simulink model "Simulator"  (R2023b)
settings: Solver=ode5  StartTime=0.0  StopTime=time.value/15/24  FixedStep=clock.sampleTime.value  RelTol=1e-11  AbsTol=1e-12
undefined symbols (not defined in the file or in its folder): aging_clock, attitude, bias_clock, bias_gyro, chi2inv, clock, drift_clock, Environment, IMU, IMU_filter, Propagation, R_sensor2body, starTracker, vb, vm, x0, xb, xm
libraries: matrix_library x11, sensors_subsystems x4, nav_lib x3, aerolibutil x2, dyn_lib x1, simulink x1
settings Model: DataDictionary=SimulationDict.sldd  EnableAccessToBaseWorkspace=off  SimulationMode=accelerator  Creator=brent  LastModifiedBy=brent
settings SolverCC: MinimalZcImpactIntegration=on
settings DebuggingCC: ReadBeforeWriteMsg=DisableAll  WriteAfterWriteMsg=DisableAll  WriteAfterReadMsg=DisableAll  MultiTaskDSMMsg=none
settings ModelReferenceCC: UpdateModelReferenceTargets=IfOutOfDate
settings SFSimCC: SFSimEcho=off
settings RTWCC: BuildConfiguration=Faster Runs

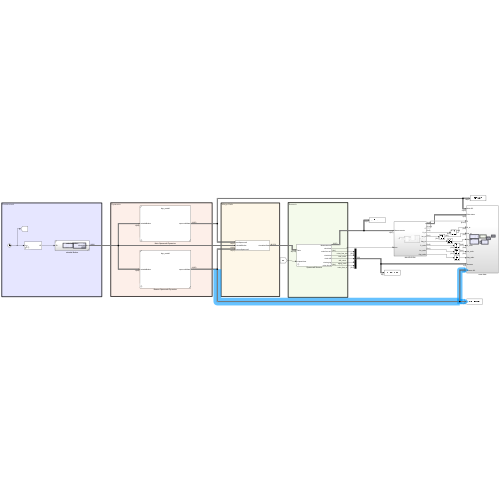
[thumbnail: Simulink's stored preview of the top-level diagram]
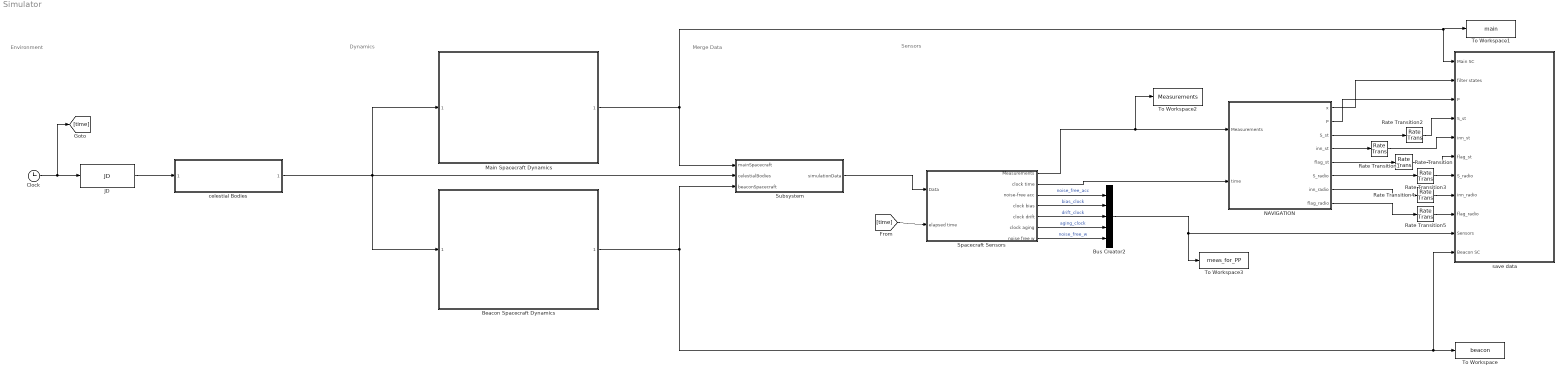
== system Simulator ==
  note: Sensors
  note: Merge Data
  note: Dynamics
  note: Environment
  Beacon Spacecraft Dynamics : Subsystem  ReferencedSubsystem=dyn_model  Environment=Environment  Spacecraft=BeaconSpacecraft  sc_type="\"beacon\""
  Bus Creator2 : BusCreator  Inputs=5
  Clock : Clock
  JD : dyn_lib/JD  year=Environment.Date.year  month=Environment.Date.month  day=Environment.Date.day  hour=Environment.Date.hour  min=Environment.Date.min  sec=Environment.Date.sec
      settings: SourceProductName=Dynamics library
  Main Spacecraft Dynamics : Subsystem  ReferencedSubsystem=dyn_model  Environment=Environment  Spacecraft=MainSpacecraft  sc_type="\"main\""
  NAVIGATION : Subsystem
  Rate Transition{,1..5} (6 alike) : RateTransition  OutPortSampleTime=1/Propagation.lf.value
  Spacecraft Sensors : Subsystem
      mask DialogControl DescGroupVar Prompt: Main spacecraft sensors
  Subsystem : Subsystem
  To Workspace : ToWorkspace  VariableName=beacon  SaveFormat=Timeseries  SampleTime=-1
  To Workspace1 : ToWorkspace  VariableName=main  SaveFormat=Timeseries  SampleTime=-1
  To Workspace2 : ToWorkspace  VariableName=Measurements  SaveFormat=Timeseries  SampleTime=-1
  To Workspace3 : ToWorkspace  VariableName=meas_for_PP  SaveFormat=Timeseries  SampleTime=-1
  celestial Bodies : Subsystem  ReferencedSubsystem=celestialBodies
      settings: PermitHierarchicalResolution=None
  save data : Subsystem
  wires:
  JD/1 -> celestial Bodies/1
  Clock/1 -> [time], JD/1
  celestial Bodies/1 -> Main Spacecraft Dynamics/1, Subsystem/2(celestialBodies), Beacon Spacecraft Dynamics/1
  Subsystem/1(simulationData) -> Spacecraft Sensors/1(Data)
  [time] -> Spacecraft Sensors/2(elapsed time)
  NAVIGATION/1(x) -> save data/2(filter states)
  Spacecraft Sensors/2(clock time) -> NAVIGATION/2(time)
  Spacecraft Sensors/1(Measurements) -> To Workspace2/1, NAVIGATION/1(Measurements)
  Main Spacecraft Dynamics/1 -> Subsystem/1(mainSpacecraft), save data/1(Main SC), To Workspace1/1
  Beacon Spacecraft Dynamics/1 -> To Workspace/1, save data/11(Beacon SC), Subsystem/3(beaconSpacecraft)
  Spacecraft Sensors/4(clock bias) -> Bus Creator2/2  "bias_clock"
  Spacecraft Sensors/5(clock drift) -> Bus Creator2/3  "drift_clock"
  Spacecraft Sensors/3(noise-free acc) -> Bus Creator2/1  "noise_free_acc"
  Spacecraft Sensors/6(clock aging) -> Bus Creator2/4  "aging_clock"
  Spacecraft Sensors/7(noise free w) -> Bus Creator2/5  "noise_free_w"
  Bus Creator2/1 -> To Workspace3/1, save data/10(Sensors)
  NAVIGATION/2(P) -> save data/3(P)
  NAVIGATION/3(S_st) -> Rate Transition2/1
  NAVIGATION/4(inn_st) -> Rate Transition1/1
  NAVIGATION/5(flag_st) -> Rate Transition/1
  Rate Transition/1 -> save data/6(flag_st)
  Rate Transition1/1 -> save data/5(inn_st)
  Rate Transition2/1 -> save data/4(S_st)
  NAVIGATION/6(S_radio) -> Rate Transition3/1
  NAVIGATION/7(inn_radio) -> Rate Transition4/1
  NAVIGATION/8(flag_radio) -> Rate Transition5/1
  Rate Transition3/1 -> save data/7(S_radio)
  Rate Transition4/1 -> save data/8(inn_radio)
  Rate Transition5/1 -> save data/9(flag_radio)

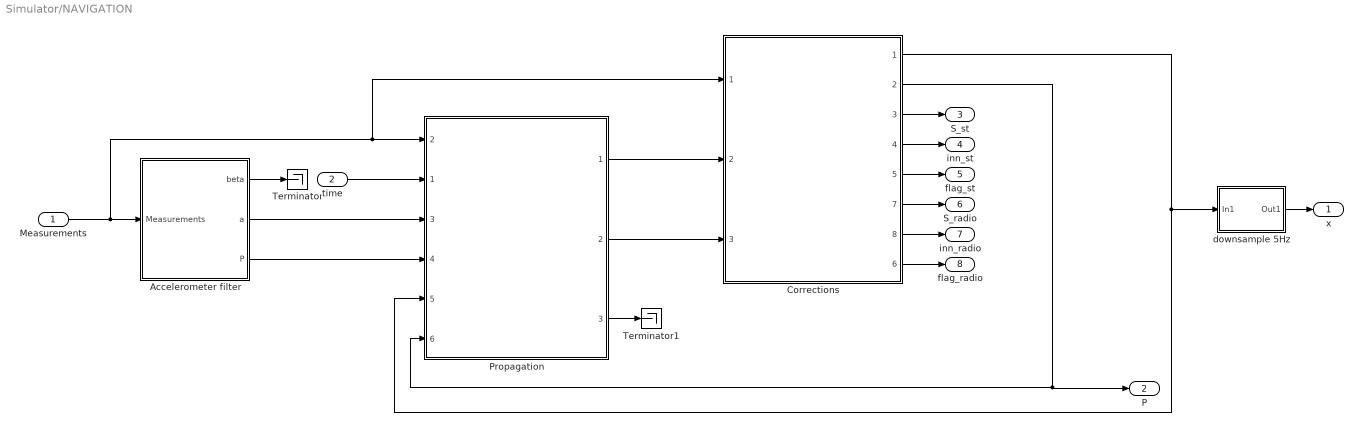
== system Simulator/NAVIGATION ==
  Measurements : Inport
  time : Inport  Port=2
  Accelerometer filter : Subsystem
  Corrections : Subsystem  SystemSampleTime=1/Propagation.lf.value  ReferencedSubsystem=Corrections
      settings: PortSchema="{\"entries\":[{\"content\":{\"sides\":[{\"content\":{\"connectorIds\":[\"In1\",\"In2\",\"In3\"]},\"type\":\"ConnectorPlacement.EquallySpacedRectSide\",\"uuid\":\"4a0e20b6-6862-4fa1-a2e9-6e1d8bf74bd7\"},{\"content\":{\"connectorIds\":[\"Out1\",\"Out2\",\"Out3\",\"Out4\",\"Out5\",\"Out7\",\"Out8\",\"Out6\"],\"side\":\"RIGHT\"},\"type\":\"ConnectorPlacement.EquallySpacedRectSide\",\"uuid\":\"f2385953-66e1-45ae-9533-3c9604da3d88\"},{\"content\":{\"side\":\"TOP\"},\"type\":\"ConnectorPlacement.EquallySpacedRectSide\",\"uuid\":\"afdba90b-0ddf-41f8-b327-cae45893fc5e\"}]},\"type\":\"ConnectorPlacement.EquallySpacedConnector\",\"uuid\":\"034f2023-7f19-4627-93e0-5347c716ea57\"}],\"packageUris\":[\"http://schema.mathworks.com/mf0/Connector/R2020b\"],\"version\":\"1.0\"}"
  Propagation : Subsystem  ReferencedSubsystem=propagation
      settings: PortSchema="{\"entries\":[{\"content\":{\"sides\":[{\"content\":{\"connectorIds\":[\"In2\",\"In1\",\"In3\",\"In4\",\"In5\",\"In6\"]},\"type\":\"ConnectorPlacement.EquallySpacedRectSide\",\"uuid\":\"bbcb9a4b-74e9-4951-92cf-711ba847ce16\"},{\"content\":{\"connectorIds\":[\"Out1\",\"Out2\",\"Out3\"],\"side\":\"RIGHT\"},\"type\":\"ConnectorPlacement.EquallySpacedRectSide\",\"uuid\":\"3c0c2903-3498-4d45-863b-5de13beed929\"},{\"content\":{\"side\":\"TOP\"},\"type\":\"ConnectorPlacement.EquallySpacedRectSide\",\"uuid\":\"36c2c2d5-e434-425c-9c60-e059bfa56cb3\"}]},\"type\":\"ConnectorPlacement.EquallySpacedConnector\",\"uuid\":\"92b99c71-176e-44fa-97a0-fffc1d5455e4\"}],\"packageUris\":[\"http://schema.mathworks.com/mf0/Connector/R2020b\"],\"version\":\"1.0\"}"
  Terminator : Terminator
  Terminator1 : Terminator
  downsample 5Hz : Subsystem  TreatAsAtomicUnit=on  SystemSampleTime=1/Propagation.lf.value
  x : Outport
  P : Outport  Port=2
  S_st : Outport  Port=3
  inn_st : Outport  Port=4
  flag_st : Outport  Port=5
  S_radio : Outport  Port=6
  inn_radio : Outport  Port=7
  flag_radio : Outport  Port=8
  wires:
  time/1 -> Propagation/1
  Propagation/1 -> Corrections/2
  Propagation/2 -> Corrections/3
  Corrections/2 -> P/1, Propagation/6
  Measurements/1 -> Accelerometer filter/1(Measurements), Corrections/1, Propagation/2
  Corrections/1 -> downsample 5Hz/1(In1), Propagation/5
  Propagation/3 -> Terminator1/1
  downsample 5Hz/1(Out1) -> x/1
  Accelerometer filter/1(beta) -> Terminator/1
  Accelerometer filter/2(a) -> Propagation/3
  Accelerometer filter/3(P) -> Propagation/4
  Corrections/3 -> S_st/1
  Corrections/5 -> flag_st/1
  Corrections/4 -> inn_st/1
  Corrections/7 -> S_radio/1
  Corrections/8 -> inn_radio/1
  Corrections/6 -> flag_radio/1

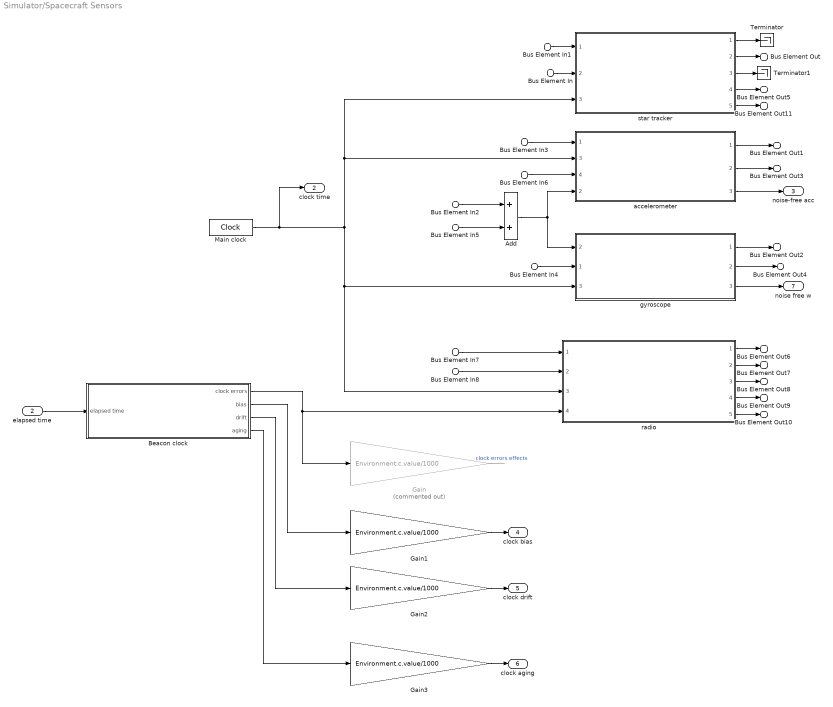
== system Simulator/Spacecraft Sensors ==
  Bus Element In1 : Inport  PortName=Data  Element=celestialBodies
  Bus Element In8 : Inport  PortName=Data  Element=beaconSpacecraft.x
  Bus Element In : Inport  PortName=Data  Element=mainSpacecraft
  Bus Element In7 : Inport  PortName=Data  Element=mainSpacecraft.x
  Bus Element In3 : Inport  PortName=Data  Element=mainSpacecraft.w
  Bus Element In4 : Inport  PortName=Data  Element=mainSpacecraft.w
  Bus Element In6 : Inport  PortName=Data  Element=mainSpacecraft.q
  Bus Element In2 : Inport  PortName=Data  Element=mainSpacecraft.a.srp
  Bus Element In5 : Inport  PortName=Data  Element=mainSpacecraft.a.thrust
  elapsed time : Inport  Port=2
  " Beacon clock" : Subsystem  TreatAsAtomicUnit=on  SystemSampleTime=clock.sampleTime.value
  Add : Sum
  Gain : Gain  Commented=on  Gain=Environment.c.value/1000
  Gain1 : Gain  Gain=Environment.c.value/1000
  Gain2 : Gain  Gain=Environment.c.value/1000
  Gain3 : Gain  Gain=Environment.c.value/1000
  Main clock : DigitalClock  SampleTime=clock.sampleTime.value
  Terminator : Terminator
  Terminator1 : Terminator
  accelerometer : Subsystem  TreatAsAtomicUnit=on  SystemSampleTime=IMU.accelerometer.sampleTime.value  ReferencedSubsystem=accelerometer
      settings: PortSchema="{\"entries\":[{\"content\":{\"sides\":[{\"content\":{\"connectorIds\":[\"In1\",\"In3\",\"In4\",\"In2\"]},\"type\":\"ConnectorPlacement.EquallySpacedRectSide\",\"uuid\":\"f690aca1-0f02-47fc-8596-4493e25f285c\"},{\"content\":{\"connectorIds\":[\"Out1\",\"Out2\",\"Out3\"],\"side\":\"RIGHT\"},\"type\":\"ConnectorPlacement.EquallySpacedRectSide\",\"uuid\":\"ecd25334-8389-4aa4-af3e-65bbeaac2b4b\"},{\"content\":{\"side\":\"TOP\"},\"type\":\"ConnectorPlacement.EquallySpacedRectSide\",\"uuid\":\"886a7907-fe4b-4c0c-bdd8-227e17cf6450\"}]},\"type\":\"ConnectorPlacement.EquallySpacedConnector\",\"uuid\":\"5845c284-1d3d-44f6-9189-c640147e7586\"}],\"packageUris\":[\"http://schema.mathworks.com/mf0/Connector/R2020b\"],\"version\":\"1.0\"}"
  gyroscope : Subsystem  TreatAsAtomicUnit=on  SystemSampleTime=IMU.gyroscope.sampleTime.value  ReferencedSubsystem=gyroscope
      settings: PortSchema="{\"entries\":[{\"content\":{\"sides\":[{\"content\":{\"connectorIds\":[\"In2\",\"In1\",\"In3\"]},\"type\":\"ConnectorPlacement.EquallySpacedRectSide\",\"uuid\":\"a73d9eac-a576-4678-b54d-8c746de67cbf\"},{\"content\":{\"connectorIds\":[\"Out1\",\"Out2\",\"Out3\"],\"side\":\"RIGHT\"},\"type\":\"ConnectorPlacement.EquallySpacedRectSide\",\"uuid\":\"2006f466-e486-45ed-9fae-d2b9dd284ae8\"},{\"content\":{\"side\":\"TOP\"},\"type\":\"ConnectorPlacement.EquallySpacedRectSide\",\"uuid\":\"4ee25c93-8ca3-4de1-922d-e3f5ca258a10\"}]},\"type\":\"ConnectorPlacement.EquallySpacedConnector\",\"uuid\":\"108469a1-96df-4a10-b09a-846939a8a3ce\"}],\"packageUris\":[\"http://schema.mathworks.com/mf0/Connector/R2020b\"],\"version\":\"1.0\"}"
  radio : Subsystem  ReferencedSubsystem=radio
  star tracker : Subsystem  TreatAsAtomicUnit=on  SystemSampleTime=starTracker.sampleTime.value  ReferencedSubsystem=starTracker
      settings: PermitHierarchicalResolution=None
  Bus Element Out7 : Outport  PortName=Measurements  Element=radio.range_PN
  Bus Element Out6 : Outport  PortName=Measurements  Element=radio.range_CP
  Bus Element Out9 : Outport  PortName=Measurements  Element=radio.range_rate
  Bus Element Out8 : Outport  PortName=Measurements  Element=radio.range_timestamp
  Bus Element Out10 : Outport  PortName=Measurements  Element=radio.range_rate_timestamp
  Bus Element Out3 : Outport  PortName=Measurements  Element=IMU.acc_timestamp
  Bus Element Out4 : Outport  PortName=Measurements  Element=IMU.gyro_timestamp
  Bus Element Out1 : Outport  PortName=Measurements  Element=IMU.acc
  Bus Element Out2 : Outport  PortName=Measurements  Element=IMU.gyro
  Bus Element Out11 : Outport  PortName=Measurements  Element=starTracker.P_qq
  Bus Element Out5 : Outport  PortName=Measurements  Element=starTracker.timestamp
  Bus Element Out : Outport  PortName=Measurements  Element=starTracker.quaternion
  clock time : Outport  Port=2
  noise-free acc : Outport  Port=3
  clock bias : Outport  Port=4
  clock drift : Outport  Port=5
  clock aging : Outport  Port=6
  noise free w : Outport  Port=7
  wires:
  Bus Element In1/1 -> star tracker/1
  Bus Element In/1 -> star tracker/2
  star tracker/1 -> Terminator/1
  star tracker/2 -> Bus Element Out/1
  Bus Element In3/1 -> accelerometer/1
  Bus Element In4/1 -> gyroscope/1
  elapsed time/1 -> " Beacon clock"/1(elapsed time)
  star tracker/4 -> Bus Element Out5/1
  Bus Element In6/1 -> accelerometer/4
  Bus Element In7/1 -> radio/1
  Bus Element In8/1 -> radio/2
  radio/1 -> Bus Element Out6/1
  radio/2 -> Bus Element Out7/1
  radio/3 -> Bus Element Out8/1
  radio/4 -> Bus Element Out9/1
  radio/5 -> Bus Element Out10/1
  Main clock/1 -> clock time/1, star tracker/3, accelerometer/3, radio/3, gyroscope/3
  Bus Element In2/1 -> Add/1
  Bus Element In5/1 -> Add/2
  Add/1 -> gyroscope/2, accelerometer/2
  accelerometer/2 -> Bus Element Out3/1
  accelerometer/1 -> Bus Element Out1/1
  gyroscope/2 -> Bus Element Out4/1
  gyroscope/1 -> Bus Element Out2/1
  star tracker/3 -> Terminator1/1
  gyroscope/3 -> noise free w/1
  accelerometer/3 -> noise-free acc/1
  " Beacon clock"/1(clock errors) -> Gain/1, radio/4
  Gain/1 -> ?  "clock errors effects"
  Gain1/1 -> clock bias/1
  Gain2/1 -> clock drift/1
  " Beacon clock"/2(bias) -> Gain1/1
  " Beacon clock"/3(drift) -> Gain2/1
  Gain3/1 -> clock aging/1
  " Beacon clock"/4(aging) -> Gain3/1
  star tracker/5 -> Bus Element Out11/1

== system Simulator/Subsystem ==
  Bus Element In1 : Inport  PortName=mainSpacecraft
  Bus Element In : Inport  Port=2  PortName=celestialBodies
  Bus Element In2 : Inport  Port=3  PortName=beaconSpacecraft
  Bus Element Out : Outport  PortName=simulationData  Element=celestialBodies
  Bus Element Out2 : Outport  PortName=simulationData  Element=beaconSpacecraft
  Bus Element Out1 : Outport  PortName=simulationData  Element=mainSpacecraft
  wires:
  Bus Element In/1 -> Bus Element Out/1
  Bus Element In1/1 -> Bus Element Out1/1
  Bus Element In2/1 -> Bus Element Out2/1

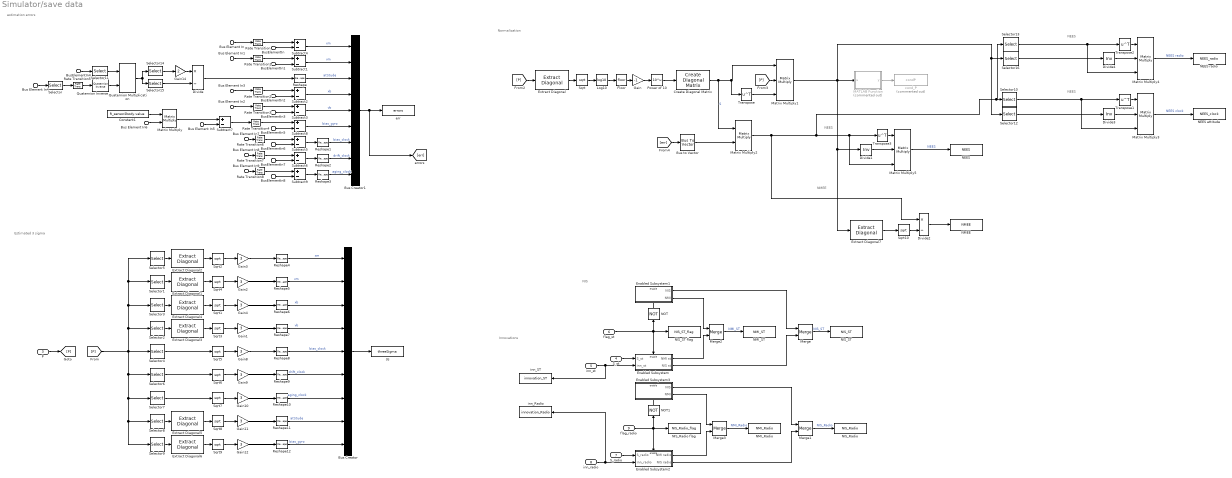
== system Simulator/save data ==
  note: Innovations
  note: NIS
  note: NMEE
  note: Normalization
  note: NEES
  note: Estimated 3 sigma
  note: estimation errors
  note: NEES
  note: NEES
  Bus Element In : Inport  PortName=Main SC  Element=x
  Bus Element In1 : Inport  PortName=Main SC  Element=v
  Bus Element In5 : Inport  PortName=Main SC  Element=w
  Bus Element In4 : Inport  PortName=Main SC  Element=q
  BusElementIn : Inport  Port=2  PortName=filter states  Element=x_m
  BusElementIn1 : Inport  Port=2  PortName=filter states  Element=v_m
  BusElementIn4 : Inport  Port=2  PortName=filter states  Element=q_m
  BusElementIn2 : Inport  Port=2  PortName=filter states  Element=x_b
  BusElementIn3 : Inport  Port=2  PortName=filter states  Element=v_b
  BusElementIn5 : Inport  Port=2  PortName=filter states  Element=bias_gyro
  BusElementIn6 : Inport  Port=2  PortName=filter states  Element=bias_clock
  BusElementIn7 : Inport  Port=2  PortName=filter states  Element=drift_clock
  BusElementIn8 : Inport  Port=2  PortName=filter states  Element=aging_clock
  P : Inport  Port=3
  S_st : Inport  Port=4
  inn_st : Inport  Port=5
  flag_st : Inport  Port=6
  S_radio : Inport  Port=7
  inn_radio : Inport  Port=8
  flag_radio : Inport  Port=9
  Bus Element In6 : Inport  Port=10  PortName=Sensors  Element=noise_free_w
  Bus Element In7 : Inport  Port=10  PortName=Sensors  Element=bias_clock
  Bus Element In8 : Inport  Port=10  PortName=Sensors  Element=drift_clock
  Bus Element In9 : Inport  Port=10  PortName=Sensors  Element=aging_clock
  Bus Element In3 : Inport  Port=11  PortName=Beacon SC  Element=x
  Bus Element In2 : Inport  Port=11  PortName=Beacon SC  Element=v
  3s : ToWorkspace  VariableName=threeSigma  SaveFormat=Timeseries  SampleTime=-1
  Bus Creator : BusCreator  Inputs=xm,vm,xb,vb,bias_clock,drift_clock,aging_clock,attitude,bias_gyro
  Bus Creator1 : BusCreator  Inputs=9
  Bus to Vector : BusToVector
  Constant1 : Constant  Value=R_sensor2body.value
  Create Diagonal Matrix : matrix_library/Create Diagonal Matrix
      settings: LibrarySourceBlock=|
      | simulink/Matrix
      | Operations/Create Diagonal
      | Matrix
  Divide : Product  Inputs=*/
  Divide1 : Product  Inputs=/  Multiplication=Matrix(*)
  Divide2 : Product  Inputs=*/
  Divide3 : Product  Inputs=/  Multiplication=Matrix(*)
  Divide4 : Product  Inputs=/  Multiplication=Matrix(*)
  Enabled Subsystem : Subsystem  TreatAsAtomicUnit=on
  Enabled Subsystem1 : Subsystem  TreatAsAtomicUnit=on
  Enabled Subsystem2 : Subsystem  TreatAsAtomicUnit=on
  Enabled Subsystem3 : Subsystem  TreatAsAtomicUnit=on
  Extract Diagonal{,1..7} (8 alike) : matrix_library/Extract Diagonal
      settings: LibrarySourceBlock=|
      | simulink/Matrix
      | Operations/Extract Diagonal
  Floor : Rounding
  Gain : Gain  Gain=-1
  Gain{1..4,8..12} (9 alike) : Gain  Gain=3
  Gain14 : Gain  Gain=2
  Log10 : Math  Operator=log10
  MATLAB Function : MATLAB Function  Commented=on  TreatAsAtomicUnit=on
  Matrix Multiply : Product  Multiplication=Matrix(*)
  Matrix Multiply{1,3..5} (4 alike) : Product  Inputs=3  Multiplication=Matrix(*)
  Matrix Multiply2 : Product  Multiplication=Matrix(*)
  Merge{,1..3} (4 alike) : Merge
  NEES : ToWorkspace  VariableName=NEES  SaveFormat=Timeseries  SampleTime=-1
  NEES attitude : ToWorkspace  VariableName=NEES_clock  SaveFormat=Timeseries  SampleTime=-1
  NEES radio : ToWorkspace  VariableName=NEES_radio  SaveFormat=Timeseries  SampleTime=-1
  NIS_Radio : ToWorkspace  VariableName=NIS_Radio  SaveFormat=Timeseries  SampleTime=-1
  NIS_Radio flag : ToWorkspace  VariableName=NIS_Radio_flag  SaveFormat=Timeseries  SampleTime=-1
  NIS_ST : ToWorkspace  VariableName=NIS_ST  SaveFormat=Timeseries  SampleTime=-1
  NIS_ST flag : ToWorkspace  VariableName=NIS_ST_flag  SaveFormat=Timeseries  SampleTime=-1
  NMEE : ToWorkspace  VariableName=NMEE  SaveFormat=Timeseries  SampleTime=-1
  NMI_Radio : ToWorkspace  VariableName=NMI_Radio  SaveFormat=Timeseries  SampleTime=-1
  NMI_ST : ToWorkspace  VariableName=NMI_ST  SaveFormat=Timeseries  SampleTime=-1
  NOT : Logic  Operator=NOT  IconShape=distinctive  AllPortsSameDT=off  OutDataTypeStr=boolean
  NOT1 : Logic  Operator=NOT  IconShape=distinctive  AllPortsSameDT=off  OutDataTypeStr=boolean
  Power of 10 : Math  Operator=10^u
  Quaternion Inverse : aerolibutil/Quaternion Inverse
  Quaternion Multiplication : aerolibutil/Quaternion Multiplication
  Rate Transition{,1..8} (9 alike) : RateTransition  OutPortSampleTime=1/Propagation.lf.value
  Reshape{,1..12} (13 alike) : Reshape  OutputDimensionality=Column vector (2-D)
  Selector : Selector  InputPortWidth=4  IndexOptions=Index vector (dialog)  Indices=[4 1 2 3]  OutputSizes=1
  Selector1 : Selector  NumberOfDimensions=2  InputPortWidth=3  IndexOptions=Index vector (dialog),Index vector (dialog)  Indices=4:6,4:6  OutputSizes=1,1
  Selector10 : Selector  NumberOfDimensions=2  InputPortWidth=3  IndexOptions=Index vector (dialog),Select all  Indices=19:21,1  OutputSizes=1,1
  Selector11 : Selector  InputPortWidth=4  IndexOptions=Index vector (dialog)  Indices=[4 1:3]  OutputSizes=1
  Selector12 : Selector  NumberOfDimensions=2  InputPortWidth=3  IndexOptions=Index vector (dialog),Index vector (dialog)  Indices=19:21,19:21  OutputSizes=1,1
  Selector13 : Selector  NumberOfDimensions=2  InputPortWidth=3  IndexOptions=Index vector (dialog),Select all  Indices=[1:6 10:15 19:21],1  OutputSizes=1,1
  Selector14 : Selector  InputPortWidth=4  IndexOptions=Index vector (dialog)  Indices=2:4  OutputSizes=1
  Selector15 : Selector  InputPortWidth=4  IndexOptions=Index vector (dialog)  Indices=1  OutputSizes=1
  Selector16 : Selector  NumberOfDimensions=2  InputPortWidth=3  IndexOptions=Index vector (dialog),Index vector (dialog)  Indices=[1:6 10:15 19:21],[1:6 10:15 19:21]  OutputSizes=1,1
  Selector2 : Selector  NumberOfDimensions=2  InputPortWidth=3  IndexOptions=Index vector (dialog),Index vector (dialog)  Indices=13:15,13:15  OutputSizes=1,1
  Selector3 : Selector  NumberOfDimensions=2  InputPortWidth=3  IndexOptions=Index vector (dialog),Index vector (dialog)  Indices=10:12,10:12  OutputSizes=1,1
  Selector4 : Selector  NumberOfDimensions=2  InputPortWidth=3  IndexOptions=Index vector (dialog),Index vector (dialog)  Indices=19,19  OutputSizes=1,1
  Selector5 : Selector  NumberOfDimensions=2  InputPortWidth=3  IndexOptions=Index vector (dialog),Index vector (dialog)  Indices=1:3,1:3  OutputSizes=1,1
  Selector6 : Selector  NumberOfDimensions=2  InputPortWidth=3  IndexOptions=Index vector (dialog),Index vector (dialog)  Indices=20,20  OutputSizes=1,1
  Selector7 : Selector  NumberOfDimensions=2  InputPortWidth=3  IndexOptions=Index vector (dialog),Index vector (dialog)  Indices=21,21  OutputSizes=1,1
  Selector8 : Selector  NumberOfDimensions=2  InputPortWidth=3  IndexOptions=Index vector (dialog),Index vector (dialog)  Indices=7:9,7:9  OutputSizes=1,1
  Selector9 : Selector  NumberOfDimensions=2  InputPortWidth=3  IndexOptions=Index vector (dialog),Index vector (dialog)  Indices=16:18,16:18  OutputSizes=1,1
  Sqrt{,1..10} (11 alike) : Sqrt
  Subtract{1..9} (9 alike) : Sum  Inputs=+-
  Transpose{,1..3} (4 alike) : Math  Operator=transpose
  cond_P : ToWorkspace  Commented=on  VariableName=condP  SaveFormat=Timeseries  SampleTime=-1
  err : ToWorkspace  VariableName=errors  SaveFormat=Timeseries  SampleTime=-1
  inn_Radio : ToWorkspace  VariableName=innovation_Radio  SaveFormat=Timeseries  SampleTime=-1
  inn_ST : ToWorkspace  VariableName=innovation_ST  SaveFormat=Timeseries  SampleTime=-1
  wires:
  Subtract4/1 -> Bus Creator1/1  "xm"
  Subtract5/1 -> Reshape1/1
  Subtract6/1 -> Reshape2/1
  Subtract9/1 -> Reshape3/1
  Subtract2/1 -> Bus Creator1/4  "xb"
  Bus Creator1/1 -> [err], err/1
  Subtract1/1 -> Bus Creator1/2  "vm"
  BusElementIn3/1 -> Subtract3/2
  Rate Transition1/1 -> Subtract1/1
  Subtract3/1 -> Bus Creator1/5  "vb"
  BusElementIn2/1 -> Subtract2/2
  BusElementIn1/1 -> Subtract1/2
  Bus Element In/1 -> Rate Transition/1
  Rate Transition2/1 -> Subtract2/1
  Rate Transition3/1 -> Subtract3/1
  Bus Element In1/1 -> Rate Transition1/1
  Bus Element In2/1 -> Rate Transition3/1
  BusElementIn/1 -> Subtract4/2
  Rate Transition/1 -> Subtract4/1
  Bus Element In3/1 -> Rate Transition2/1
  Rate Transition5/1 -> Quaternion Inverse/1
  Selector15/1 -> Divide/2
  Quaternion Inverse/1 -> Quaternion Multiplication/2
  Bus Element In4/1 -> Selector/1
  Selector14/1 -> Gain14/1
  Selector11/1 -> Quaternion Multiplication/1
  Gain14/1 -> Divide/1
  Selector/1 -> Rate Transition5/1
  BusElementIn4/1 -> Selector11/1
  Quaternion Multiplication/1 -> Selector15/1, Selector14/1
  Constant1/1 -> Matrix Multiply/1
  Matrix Multiply/1 -> Subtract7/1
  Subtract7/1 -> Rate Transition4/1
  Bus Element In5/1 -> Subtract7/2
  Subtract8/1 -> Bus Creator1/6  "bias_gyro"
  Bus Element In6/1 -> Matrix Multiply/2
  BusElementIn6/1 -> Subtract5/2
  BusElementIn7/1 -> Subtract6/2
  BusElementIn8/1 -> Subtract9/2
  Bus Element In7/1 -> Rate Transition6/1
  Bus Element In8/1 -> Rate Transition7/1
  Bus Element In9/1 -> Rate Transition8/1
  Rate Transition6/1 -> Subtract5/1
  Rate Transition7/1 -> Subtract6/1
  Rate Transition8/1 -> Subtract9/1
  Rate Transition4/1 -> Subtract8/1
  BusElementIn5/1 -> Subtract8/2
  Sqrt6/1 -> Gain9/1
  Extract Diagonal1/1 -> Sqrt4/1
  Gain2/1 -> Reshape5/1
  Gain12/1 -> Reshape12/1
  Selector8/1 -> Extract Diagonal5/1
  Gain4/1 -> Reshape6/1
  Sqrt7/1 -> Gain10/1
  Extract Diagonal2/1 -> Sqrt2/1
  Extract Diagonal6/1 -> Sqrt9/1
  Gain10/1 -> Reshape10/1
  Selector6/1 -> Sqrt6/1
  Selector1/1 -> Extract Diagonal1/1
  Selector7/1 -> Sqrt7/1
  Sqrt8/1 -> Gain11/1
  Extract Diagonal4/1 -> Sqrt1/1
  Gain1/1 -> Reshape7/1
  Sqrt1/1 -> Gain4/1
  Sqrt4/1 -> Gain2/1
  Extract Diagonal3/1 -> Sqrt3/1
  Sqrt9/1 -> Gain12/1
  Selector2/1 -> Extract Diagonal3/1
  Selector3/1 -> Extract Diagonal4/1
  Sqrt2/1 -> Gain3/1
  Selector5/1 -> Extract Diagonal2/1
  Selector9/1 -> Extract Diagonal6/1
  Gain9/1 -> Reshape9/1
  Gain3/1 -> Reshape4/1
  Gain11/1 -> Reshape11/1
  Sqrt5/1 -> Gain8/1
  Sqrt3/1 -> Gain1/1
  Gain8/1 -> Reshape8/1
  Selector4/1 -> Sqrt5/1
  [P] -> Selector9/1, Selector8/1, Selector7/1, Selector6/1, Selector4/1, Selector2/1, Selector5/1, Selector1/1, Selector3/1
  Extract Diagonal5/1 -> Sqrt8/1
  P/1 -> [P]
  Bus Creator/1 -> 3s/1
  [P] -> Extract Diagonal/1
  Extract Diagonal/1 -> Sqrt/1
  Sqrt/1 -> Log10/1
  Log10/1 -> Floor/1
  Floor/1 -> Gain/1
  Gain/1 -> Power of 10/1
  Power of 10/1 -> Create Diagonal Matrix/1
  Create Diagonal Matrix/1 -> Matrix Multiply2/1, Transpose/1, Matrix Multiply1/1  "S"
  Transpose/1 -> Matrix Multiply1/3
  [err] -> Bus to Vector/1
  Bus to Vector/1 -> Matrix Multiply2/2
  Divide1/1 -> Matrix Multiply5/2
  Transpose3/1 -> Matrix Multiply5/1
  Matrix Multiply5/1 -> NEES/1  "NEES"
  [P] -> Matrix Multiply1/2
  Extract Diagonal7/1 -> Sqrt10/1
  Sqrt10/1 -> Divide2/2
  Divide2/1 -> NMEE/1
  MATLAB Function/1(y) -> cond_P/1
  Matrix Multiply2/1 -> Divide2/1, Selector13/1, Selector10/1, Matrix Multiply5/3, Transpose3/1
  Matrix Multiply3/1 -> NEES attitude/1  "NEES clock"
  Transpose1/1 -> Matrix Multiply3/1
  Divide3/1 -> Matrix Multiply3/2
  Divide4/1 -> Matrix Multiply4/2
  Transpose2/1 -> Matrix Multiply4/1
  Matrix Multiply4/1 -> NEES radio/1  "NEES radio"
  Selector12/1 -> Divide3/1
  Selector10/1 -> Matrix Multiply3/3, Transpose1/1
  Selector16/1 -> Divide4/1
  Selector13/1 -> Matrix Multiply4/3, Transpose2/1
  Matrix Multiply1/1 -> Extract Diagonal7/1, Divide1/1, Selector12/1, Selector16/1, MATLAB Function/1(u)
  inn_st/1 -> Enabled Subsystem/2(inn_st), inn_ST/1
  S_st/1 -> Enabled Subsystem/1(S_st)
  flag_st/1 -> Enabled Subsystem/Enable, NIS_ST flag/1, NOT/1
  NOT/1 -> Enabled Subsystem1/Enable
  Enabled Subsystem1/1(NIS) -> Merge/1
  Enabled Subsystem/2(NIS st) -> Merge/2
  Merge/1 -> NIS_ST/1  "NIS_ST"
  Enabled Subsystem2/2(NIS radio) -> Merge1/2
  Merge1/1 -> NIS_Radio/1  "NIS_Radio"
  S_radio/1 -> Enabled Subsystem2/1(S_radio)
  NOT1/1 -> Enabled Subsystem3/Enable
  flag_radio/1 -> Enabled Subsystem2/Enable, NIS_Radio flag/1, NOT1/1
  inn_radio/1 -> inn_Radio/1, Enabled Subsystem2/2(inn_radio)
  Enabled Subsystem3/1(NIS) -> Merge1/1
  Reshape/1 -> Bus Creator1/3  "attitude"
  Divide/1 -> Reshape/1
  Reshape1/1 -> Bus Creator1/7  "bias_clock"
  Reshape2/1 -> Bus Creator1/8  "drift_clock"
  Reshape3/1 -> Bus Creator1/9  "aging_clock"
  Reshape4/1 -> Bus Creator/1  "xm"
  Reshape5/1 -> Bus Creator/2  "vm"
  Reshape6/1 -> Bus Creator/3  "xb"
  Reshape7/1 -> Bus Creator/4  "vb"
  Reshape8/1 -> Bus Creator/5  "bias_clock"
  Reshape9/1 -> Bus Creator/6  "drift_clock"
  Reshape10/1 -> Bus Creator/7  "aging_clock"
  Reshape11/1 -> Bus Creator/8  "attitude"
  Reshape12/1 -> Bus Creator/9  "bias_gyro"
  Enabled Subsystem1/2(NMI) -> Merge2/1
  Enabled Subsystem/1(NMI st) -> Merge2/2
  Merge2/1 -> NMI_ST/1  "NMI_ST"
  Enabled Subsystem2/1(NMI radio) -> Merge3/2
  Enabled Subsystem3/2(NMI) -> Merge3/1
  Merge3/1 -> NMI_Radio/1  "NMI_Radio"

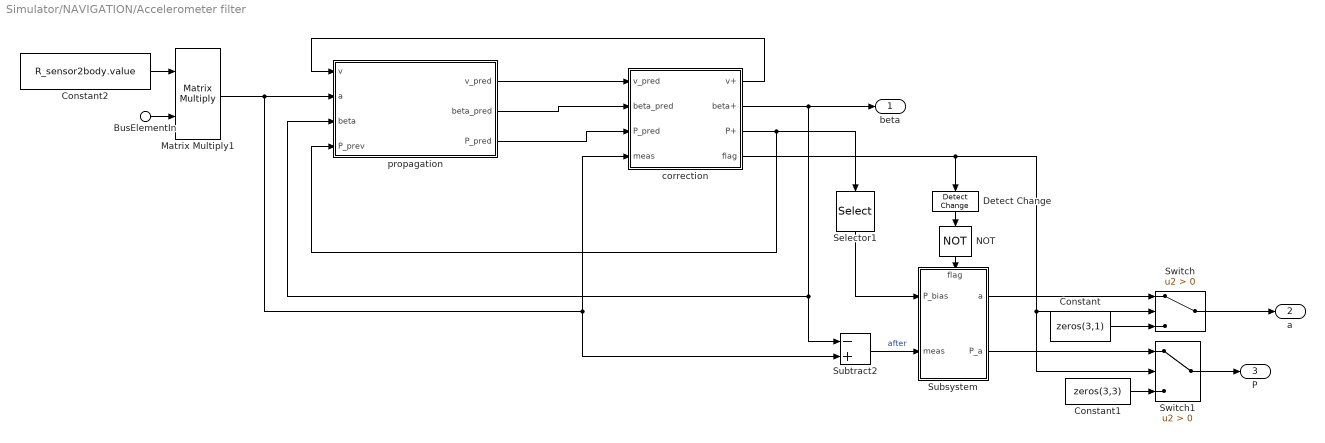
== system Simulator/NAVIGATION/Accelerometer filter ==
  BusElementIn : Inport  PortName=Measurements  Element=IMU.acc
  Constant : Constant  Value=zeros(3,1)  VectorParams1D=off
  Constant1 : Constant  Value=zeros(3,3)
  Constant2 : Constant  Value=R_sensor2body.value
  Detect Change : simulink/Logic and Bit Operations/Detect Change  vinit=0  OutDataTypeStr=boolean
  Matrix Multiply1 : Product  Multiplication=Matrix(*)
  NOT : Logic  Operator=NOT  IconShape=distinctive  AllPortsSameDT=off  OutDataTypeStr=boolean
  Selector1 : Selector  NumberOfDimensions=2  InputPortWidth=3  IndexOptions=Index vector (dialog),Index vector (dialog)  Indices=4:6,4:6  OutputSizes=1,1
  Subsystem : Subsystem
      settings: PortSchema="{\"entries\":[{\"content\":{\"sides\":[{\"content\":{\"connectorIds\":[\"In1\",\"In2\"]},\"type\":\"ConnectorPlacement.EquallySpacedRectSide\",\"uuid\":\"04984c6d-68bb-4868-b555-561b55ad66cf\"},{\"content\":{\"connectorIds\":[\"Out1\",\"Out2\"],\"side\":\"RIGHT\"},\"type\":\"ConnectorPlacement.EquallySpacedRectSide\",\"uuid\":\"a81d3184-9e13-42c8-a176-83bd8c1c8126\"},{\"content\":{\"connectorIds\":[\"In3\"],\"side\":\"TOP\"},\"type\":\"ConnectorPlacement.EquallySpacedRectSide\",\"uuid\":\"95046c64-69a7-4e42-aa3a-b7d167259f83\"}]},\"type\":\"ConnectorPlacement.EquallySpacedConnector\",\"uuid\":\"a38104d1-1e85-4f2e-aa1d-28155c2663e4\"}],\"packageUris\":[\"http://schema.mathworks.com/mf0/Connector/R2020b\"],\"version\":\"1.0\"}"
  Subtract2 : Sum  Inputs=-+
  Switch : Switch  Criteria=u2 > Threshold  SaturateOnIntegerOverflow=off  InputSameDT=off
  Switch1 : Switch  Criteria=u2 > Threshold  SaturateOnIntegerOverflow=off  InputSameDT=off
  correction : Subsystem
  propagation : Subsystem  mask{dt=IMU.accelerometer.sampleTime.value}
      mask prompts: dt "sample time"
      mask DialogControl DescGroupVar Prompt: Propagation Step
  beta : Outport
  a : Outport  Port=2
  P : Outport  Port=3
  wires:
  correction/2(beta+) -> beta/1, Subtract2/1, propagation/3(beta)
  propagation/2(beta_pred) -> correction/2(beta_pred)
  propagation/3(P_pred) -> correction/3(P_pred)
  propagation/1(v_pred) -> correction/1(v_pred)
  Switch/1 -> a/1
  Constant/1 -> Switch/3
  Subsystem/1(a) -> Switch/1
  Subtract2/1 -> Subsystem/2(meas)  "after"
  Matrix Multiply1/1 -> correction/4(meas), Subtract2/2, propagation/2(a)
  Detect Change/1 -> NOT/1
  NOT/1 -> Subsystem/3(flag)
  correction/3(P+) -> Selector1/1, propagation/4(P_prev)
  correction/1(v+) -> propagation/1(v)
  Subsystem/2(P_a) -> Switch1/1
  Constant1/1 -> Switch1/3
  Selector1/1 -> Subsystem/1(P_bias)
  Constant2/1 -> Matrix Multiply1/1
  BusElementIn/1 -> Matrix Multiply1/2
  correction/4(flag) -> Detect Change/1, Switch1/2, Switch/2
  Switch1/1 -> P/1

== system Simulator/NAVIGATION/downsample 5Hz ==
  In1 : Inport
  Out1 : Outport
  wires:
  In1/1 -> Out1/1

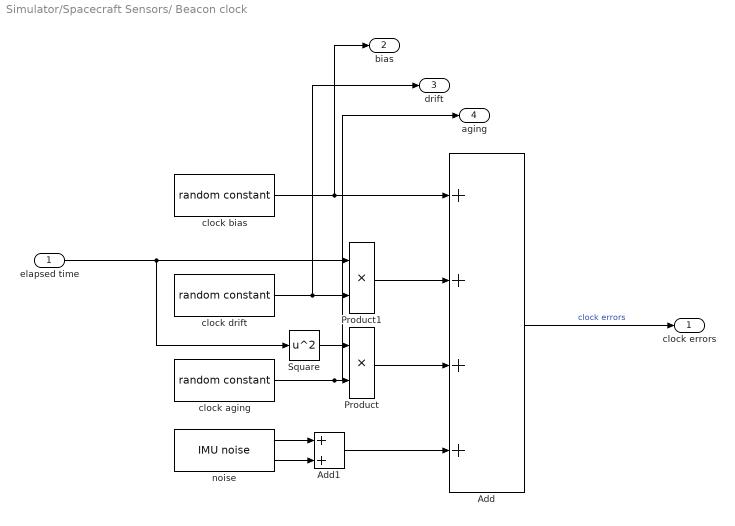
== system Simulator/Spacecraft Sensors/ Beacon clock ==
  elapsed time : Inport
  Add : Sum  Inputs=++++
  Add1 : Sum
  Product : Product
  Product1 : Product
  Square : Math  Operator=square
  clock aging : sensors_subsystems/random constant  mean=clock.deltaT2.nominal  dev=clock.deltaT2.std
      settings: SourceProductName=Sensors library
  clock bias : sensors_subsystems/random constant  mean=clock.deltaT0.nominal  dev=clock.deltaT0.std
      settings: SourceProductName=Sensors library
  clock drift : sensors_subsystems/random constant  mean=clock.deltaT1.nominal  dev=clock.deltaT1.std
      settings: SourceProductName=Sensors library
  noise : sensors_subsystems/IMU noise  data=clock  arw_seed=abs(round(randn(1)*1e4))  bi_seed=abs(round(randn(1)*1e4))  br_seed=abs(round(randn(1)*1e4))
      settings: SourceProductName=Sensors library
  clock errors : Outport
  bias : Outport  Port=2
  drift : Outport  Port=3
  aging : Outport  Port=4
  wires:
  Square/1 -> Product/1
  clock aging/1 -> aging/1, Product/2
  clock drift/1 -> drift/1, Product1/2
  Add/1 -> clock errors/1  "clock errors"
  noise/1 -> Add1/1
  noise/2 -> Add1/2
  Add1/1 -> Add/4
  Product1/1 -> Add/2
  clock bias/1 -> bias/1, Add/1
  elapsed time/1 -> Product1/1, Square/1
  Product/1 -> Add/3

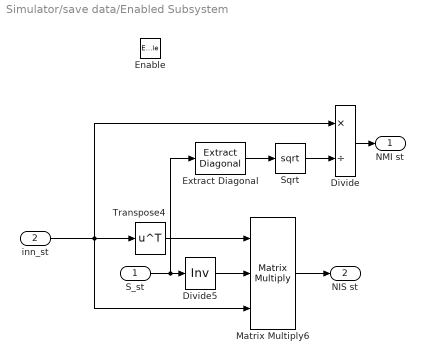
== system Simulator/save data/Enabled Subsystem ==
  S_st : Inport
  inn_st : Inport  Port=2
  Enable : EnablePort
  Divide : Product  Inputs=*/
  Divide5 : Product  Inputs=/  Multiplication=Matrix(*)
  Extract Diagonal : matrix_library/Extract Diagonal
      settings: LibrarySourceBlock=|
      | simulink/Matrix
      | Operations/Extract Diagonal
  Matrix Multiply6 : Product  Inputs=3  Multiplication=Matrix(*)
  Sqrt : Sqrt
  Transpose4 : Math  Operator=transpose
  NMI st : Outport
  NIS st : Outport  Port=2
  wires:
  Divide5/1 -> Matrix Multiply6/2
  S_st/1 -> Extract Diagonal/1, Divide5/1
  inn_st/1 -> Divide/1, Matrix Multiply6/3, Transpose4/1
  Transpose4/1 -> Matrix Multiply6/1
  Matrix Multiply6/1 -> NIS st/1
  Extract Diagonal/1 -> Sqrt/1
  Divide/1 -> NMI st/1
  Sqrt/1 -> Divide/2

== system Simulator/save data/Enabled Subsystem1 ==
  Enable : EnablePort
  Constant : Constant  Value=0
  Constant1 : Constant  Value=zeros(3,1)
  NIS : Outport
  NMI : Outport  Port=2
  wires:
  Constant/1 -> NIS/1
  Constant1/1 -> NMI/1

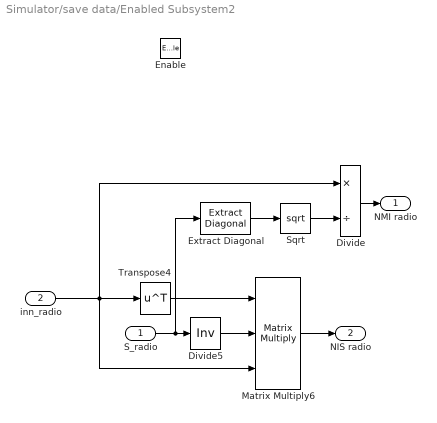
== system Simulator/save data/Enabled Subsystem2 ==
  S_radio : Inport
  inn_radio : Inport  Port=2
  Enable : EnablePort
  Divide : Product  Inputs=*/
  Divide5 : Product  Inputs=/  Multiplication=Matrix(*)
  Extract Diagonal : matrix_library/Extract Diagonal
      settings: LibrarySourceBlock=|
      | simulink/Matrix
      | Operations/Extract Diagonal
  Matrix Multiply6 : Product  Inputs=3  Multiplication=Matrix(*)
  Sqrt : Sqrt
  Transpose4 : Math  Operator=transpose
  NMI radio : Outport
  NIS radio : Outport  Port=2
  wires:
  Divide5/1 -> Matrix Multiply6/2
  Transpose4/1 -> Matrix Multiply6/1
  Matrix Multiply6/1 -> NIS radio/1
  Sqrt/1 -> Divide/2
  S_radio/1 -> Extract Diagonal/1, Divide5/1
  Extract Diagonal/1 -> Sqrt/1
  Divide/1 -> NMI radio/1
  inn_radio/1 -> Divide/1, Matrix Multiply6/3, Transpose4/1

== system Simulator/save data/Enabled Subsystem3 ==
  Enable : EnablePort
  Constant : Constant  Value=0
  Constant1 : Constant  Value=zeros(2,1)
  NIS : Outport
  NMI : Outport  Port=2
  wires:
  Constant/1 -> NIS/1
  Constant1/1 -> NMI/1

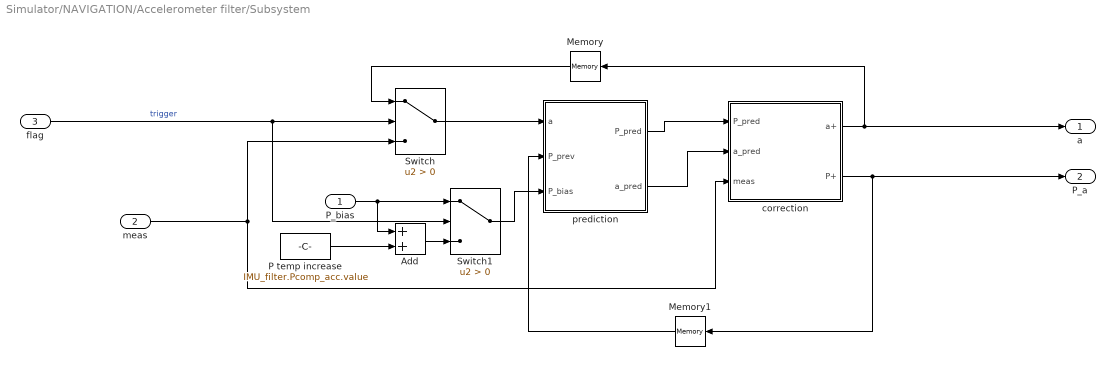
== system Simulator/NAVIGATION/Accelerometer filter/Subsystem ==
  P_bias : Inport
  meas : Inport  Port=2
  flag : Inport  Port=3
  " P temp increase" : Constant  Value=IMU_filter.Pcomp_acc.value
  Add : Sum
  Memory : Memory  InitialCondition=zeros(3,1)  InheritSampleTime=on
  Memory1 : Memory  InitialCondition=eye(3)  InheritSampleTime=on
  Switch : Switch  Criteria=u2 > Threshold  SaturateOnIntegerOverflow=off  InputSameDT=off
  Switch1 : Switch  Criteria=u2 > Threshold  SaturateOnIntegerOverflow=off  InputSameDT=off
  correction : Subsystem
  prediction : Subsystem
  a : Outport
  P_a : Outport  Port=2
  wires:
  prediction/1(P_pred) -> correction/1(P_pred)
  prediction/2(a_pred) -> correction/2(a_pred)
  correction/2(P+) -> P_a/1, Memory1/1
  Switch/1 -> prediction/1(a)
  correction/1(a+) -> Memory/1, a/1
  meas/1 -> correction/3(meas), Switch/3
  Memory/1 -> Switch/1
  flag/1 -> Switch1/2, Switch/2  "trigger"
  P_bias/1 -> Add/1, Switch1/1
  Add/1 -> Switch1/3
  " P temp increase"/1 -> Add/2
  Switch1/1 -> prediction/3(P_bias)
  Memory1/1 -> prediction/2(P_prev)

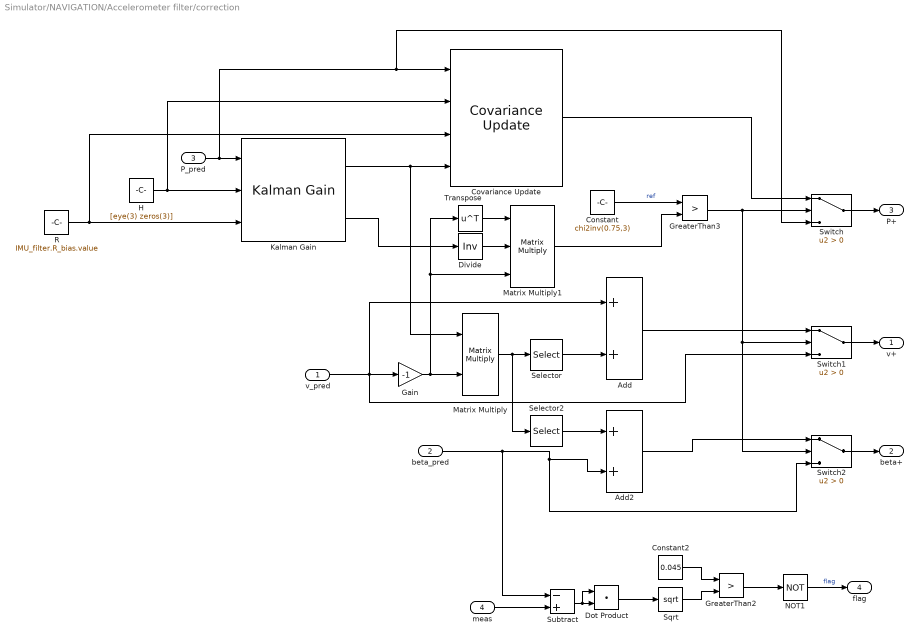
== system Simulator/NAVIGATION/Accelerometer filter/correction ==
  v_pred : Inport
  beta_pred : Inport  Port=2
  P_pred : Inport  Port=3
  meas : Inport  Port=4
  Add : Sum
  Add2 : Sum
  Constant : Constant  Value=chi2inv(0.75,3)
  Constant2 : Constant  Value=0.045
  Covariance Update : nav_lib/Covariance Update
      settings: SourceProductName=Navigation library
  Divide : Product  Inputs=/  Multiplication=Matrix(*)
  Dot Product : DotProduct  OutDataTypeStr=Inherit: Inherit via internal rule
  Gain : Gain  Gain=-1
  GreaterThan2 : RelationalOperator  Operator=>  OutDataTypeStr=boolean  RndMeth=Simplest  InputSameDT=off
  GreaterThan3 : RelationalOperator  Operator=>  OutDataTypeStr=boolean  RndMeth=Simplest  InputSameDT=off
  H : Constant  Value=[eye(3) zeros(3)]
  Kalman Gain : nav_lib/Kalman Gain
      settings: SourceProductName=Navigation library
  Matrix Multiply : Product  Multiplication=Matrix(*)
  Matrix Multiply1 : Product  Inputs=3  Multiplication=Matrix(*)
  NOT1 : Logic  Operator=NOT  IconShape=distinctive  AllPortsSameDT=off  OutDataTypeStr=boolean
  R : Constant  Value=IMU_filter.R_bias.value
  Selector : Selector  NumberOfDimensions=2  InputPortWidth=3  IndexOptions=Index vector (dialog),Select all  Indices=1:3,1  OutputSizes=1,1
  Selector2 : Selector  NumberOfDimensions=2  InputPortWidth=3  IndexOptions=Index vector (dialog),Select all  Indices=4:6,1  OutputSizes=1,1
  Sqrt : Sqrt
  Subtract : Sum  Inputs=-+
  Switch : Switch  Criteria=u2 > Threshold  SaturateOnIntegerOverflow=off  InputSameDT=off
  Switch1 : Switch  Criteria=u2 > Threshold  SaturateOnIntegerOverflow=off  InputSameDT=off
  Switch2 : Switch  Criteria=u2 > Threshold  SaturateOnIntegerOverflow=off  InputSameDT=off
  Transpose : Math  Operator=transpose
  v+ : Outport
  beta+ : Outport  Port=2
  P+ : Outport  Port=3
  flag : Outport  Port=4
  wires:
  beta_pred/1 -> Subtract/1, Switch2/3, Add2/2
  Selector2/1 -> Add2/1
  Selector/1 -> Add/2
  Matrix Multiply/1 -> Selector/1, Selector2/1
  Gain/1 -> Matrix Multiply1/3, Transpose/1, Matrix Multiply/2
  v_pred/1 -> Switch1/3, Add/1, Gain/1
  H/1 -> Kalman Gain/2, Covariance Update/2
  P_pred/1 -> Kalman Gain/1, Switch/3, Covariance Update/1
  R/1 -> Kalman Gain/3, Covariance Update/3
  Kalman Gain/1 -> Covariance Update/4, Matrix Multiply/1
  Transpose/1 -> Matrix Multiply1/1
  Divide/1 -> Matrix Multiply1/2
  Constant/1 -> GreaterThan3/1  "ref"
  Matrix Multiply1/1 -> GreaterThan3/2
  GreaterThan3/1 -> Switch/2, Switch1/2, Switch2/2
  Switch/1 -> P+/1
  Covariance Update/1 -> Switch/1
  Add/1 -> Switch1/1
  Switch1/1 -> v+/1
  Switch2/1 -> beta+/1
  Add2/1 -> Switch2/1
  Kalman Gain/2 -> Divide/1
  Sqrt/1 -> GreaterThan2/2
  Constant2/1 -> GreaterThan2/1
  GreaterThan2/1 -> NOT1/1
  Dot Product/1 -> Sqrt/1
  NOT1/1 -> flag/1  "flag"
  Subtract/1 -> Dot Product/1, Dot Product/2
  meas/1 -> Subtract/2

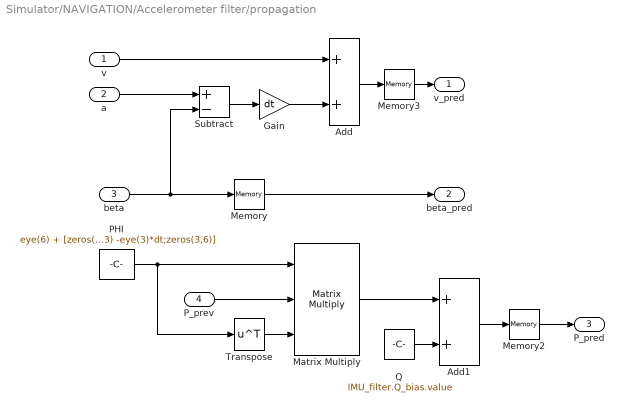
== system Simulator/NAVIGATION/Accelerometer filter/propagation ==
  v : Inport
  a : Inport  Port=2
  beta : Inport  Port=3
  P_prev : Inport  Port=4
  Add : Sum
  Add1 : Sum
  Gain : Gain  Gain=dt
  Matrix Multiply : Product  Inputs=3  Multiplication=Matrix(*)
  Memory : Memory  InitialCondition=x0.value(17:19)
  Memory2 : Memory  InitialCondition=eye(6)*1e-4
  Memory3 : Memory  InitialCondition=zeros(3,1)
  PHI : Constant  Value=eye(6) + [zeros(3) -eye(3)*dt;zeros(3,6)]
  Q : Constant  Value=IMU_filter.Q_bias.value
  Subtract : Sum  Inputs=+-
  Transpose : Math  Operator=transpose
  v_pred : Outport
  beta_pred : Outport  Port=2
  P_pred : Outport  Port=3
  wires:
  Add1/1 -> Memory2/1
  Matrix Multiply/1 -> Add1/1
  Q/1 -> Add1/2
  P_prev/1 -> Matrix Multiply/2
  Transpose/1 -> Matrix Multiply/3
  PHI/1 -> Matrix Multiply/1, Transpose/1
  Add/1 -> Memory3/1
  v/1 -> Add/1
  Gain/1 -> Add/2
  Subtract/1 -> Gain/1
  a/1 -> Subtract/1
  beta/1 -> Memory/1, Subtract/2
  Memory/1 -> beta_pred/1
  Memory3/1 -> v_pred/1
  Memory2/1 -> P_pred/1

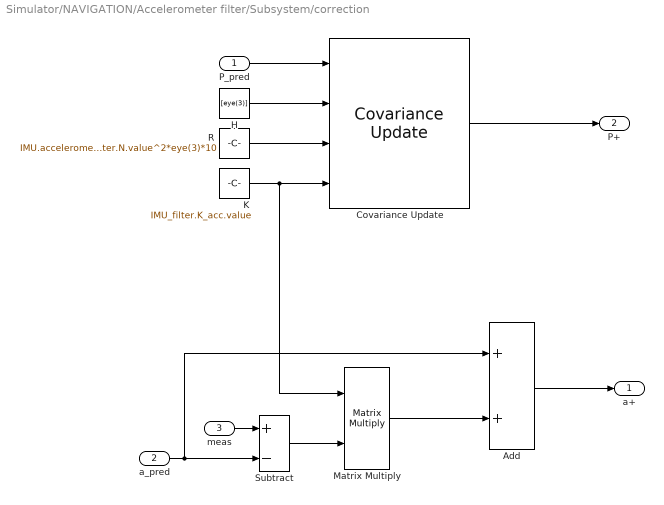
== system Simulator/NAVIGATION/Accelerometer filter/Subsystem/correction ==
  P_pred : Inport
  a_pred : Inport  Port=2
  meas : Inport  Port=3
  Add : Sum
  Covariance Update : nav_lib/Covariance Update
      settings: SourceProductName=Navigation library
  H : Constant  Value=[eye(3)]
  K : Constant  Value=IMU_filter.K_acc.value
  Matrix Multiply : Product  Multiplication=Matrix(*)
  R : Constant  Value=IMU.accelerometer.N.value^2*eye(3)*10
  Subtract : Sum  Inputs=+-
  a+ : Outport
  P+ : Outport  Port=2
  wires:
  R/1 -> Covariance Update/3
  P_pred/1 -> Covariance Update/1
  H/1 -> Covariance Update/2
  a_pred/1 -> Add/1, Subtract/2
  Subtract/1 -> Matrix Multiply/2
  Matrix Multiply/1 -> Add/2
  meas/1 -> Subtract/1
  Add/1 -> a+/1
  Covariance Update/1 -> P+/1
  K/1 -> Matrix Multiply/1, Covariance Update/4

== system Simulator/NAVIGATION/Accelerometer filter/Subsystem/prediction ==
  a : Inport
  P_prev : Inport  Port=2
  P_bias : Inport  Port=3
  Add : Sum
  Add1 : Sum
  Q : Constant  Value=IMU_filter.Q_acc.value
  P_pred : Outport
  a_pred : Outport  Port=2
  wires:
  P_prev/1 -> Add1/1
  Add1/1 -> P_pred/1
  a/1 -> a_pred/1
  Q/1 -> Add/1
  Add/1 -> Add1/2
  P_bias/1 -> Add/2

== matlab function Simulator/save data/MATLAB Function ==
  data: u input; y output
function y = fcn(u)

y = cond(u);
